simulink model "afe_abc_inv_psm_2mods"  (R2025b)
settings: Solver=ode1be  StartTime=0.0  StopTime=simlength  FixedStep=tc  MaxStep=tc
values from neighbouring files (symbols this model uses):
  n1 = 35    [voltage_islandmode_spectrum_analysis.m]    (also in voltage_spectrum_analysis.m)
undefined symbols (not defined in the file or in its folder): Adrso, afe_pwm_phase_shift_mod1, afe_pwm_phase_shift_mod2, Amplitude_U, Amplitude_V, Amplitude_W, Aresd, Bresd, Cresd, Crso, CTRPIFF_CLIP_RELEASE, dead_time_AFE, dead_time_INV, deepNEGeta, deepNEGxi, deepPOSxi, emf_fb_p, emf_fb_p_ccaller_1, emf_fb_p_ccaller_2, emf_p, emf_p_ccaller_1, emf_p_ccaller_2, end_time_LVRT, fPWM_AFE, fPWM_INV, g0_161Hz, g0_500Hz, g1_161Hz, g1_500Hz, i_grid_neg_eta_lim, i_grid_neg_eta_red_lim, i_grid_neg_xi_lim, i_grid_neg_xi_red_lim, i_grid_pos_eta_lim, i_grid_pos_eta_red_lim, ibez, id_lim, ieta_neg_ref_lim, ieta_pos_ref_lim, Igrid_phase_normalization_factor, inv_pwm_phase_shift_mod1, iq_lim, ixi_pos_ref_lim, k_frt_ref, kg, ki_afe, ki_i, ki_rc_neg_grid, ki_rc_pos_grid, ki_vs, ki_w, kp_afe, kp_i, kp_rc_neg_grid, kp_rc_pos_grid, kp_vs, kp_w, kw, l1, l2 ... (+55)
libraries: fl_lib x215, nesl_utility x107, simulink x22, cstblocks x18, threephase_inductor_lib x4, single_phase_transformer_lib x3, flexshaft_lib x1, psm x1
(part 7 of 17)

== system afe_abc_inv_psm_2mods/afe_abc_inv_psm_mod2/afe/sv_pwm/modulator1 ==
  u : Inport
  v : Inport  Port=2
  w : Inport  Port=3
  phase : Inport  Port=4
  Bus Creator : BusCreator  Inputs=3
  PWM generator : Subsystem  mask{f=fPWM_AFE, m_up=0.98, m_low=0.02, dead_time=dead_time_AFE, pos_cmd_gate=15, neg_cmd_gate=-10, polarity=1, tc=tc}
      mask prompts: f "Frequency (Hz)"; m_up "Max Input Modulation Value"; m_low "Min Input Modulation Value"; dead_time "Dead Time (s)"; pos_cmd_gate "Positive Gate Voltage (V)"; neg_cmd_gate "Negative Gate Voltage (V)"; polarity "Polarity (pu)"; tc "Sampling time"
  gate_cmds : Outport
  tag scope: TRGO_afe_module_2=global
  wires:
  PWM generator/2(gate_cmds) -> gate_cmds/1
  phase/1 -> PWM generator/2(phase)
  w/1 -> Bus Creator/3
  v/1 -> Bus Creator/2
  u/1 -> Bus Creator/1
  PWM generator/1(trgo) -> [TRGO_afe_module_2]
  Bus Creator/1 -> PWM generator/3(m_uvw())
  [time_afe_module_2] -> PWM generator/1(time_source)

== system afe_abc_inv_psm_2mods/afe_abc_inv_psm_mod2/inverter/inverter/sv_pwm ==
  duties_uvw : Inport
  Bus Selector2 : BusSelector  OutputSignals=du(k),dv(k),dw(k)
  Constant1 : Constant  Value=inv_pwm_phase_shift_mod1
  modulator1 : Subsystem
  td2tc_1 : TransferFcn  Denominator=[tc 1]
  td2tc_2 : TransferFcn  Denominator=[tc 1]
  td2tc_3 : TransferFcn  Denominator=[tc 1]
  gate_cmds : Outport
  wires:
  td2tc_2/1 -> modulator1/2(v)  "dv(t)"
  td2tc_3/1 -> modulator1/3(w)  "dw(t)"
  td2tc_1/1 -> modulator1/1(u)  "du(t)"
  duties_uvw/1 -> Bus Selector2/1
  Bus Selector2/3 -> td2tc_3/1  "<dw(k)>"
  Bus Selector2/2 -> td2tc_2/1  "<dv(k)>"
  Bus Selector2/1 -> td2tc_1/1  "<du(k)>"
  Constant1/1 -> modulator1/4(phase)
  modulator1/1(gate_cmds) -> gate_cmds/1

== system afe_abc_inv_psm_2mods/afe_abc_inv_psm_mod2/inverter/inverter/switch_1 ==
  Diode : fl_lib/Electrical/Electrical Elements/Diode  Vf=Vgamma V  Ron=Ron Ohm  Goff=1e-8 1/Ohm  i_specify=off  i_priority=None  i=0 A  i_nominal_specify=off  i_nominal_value=1  i_nominal_unit=A  v_specify=off  v_priority=None  v=0 V  v_nominal_specify=off  v_nominal_value=1  v_nominal_unit=V
  Switch : fl_lib/Electrical/Electrical Elements/Switch  R_closed=Ron Ohm  G_open=1e-8 1/Ohm  Threshold=7.5  i_specify=off  i_priority=None  i=0 A  i_nominal_specify=off  i_nominal_value=1  i_nominal_unit=A  v_specify=off  v_priority=None  v=0 V  v_nominal_specify=off  v_nominal_value=1  v_nominal_unit=V
  snubber : fl_lib/Electrical/Electrical Elements/Capacitor  c=Csnubber F  r=Rsnubber Ohm  g=0 1/Ohm  i_specify=off  i_priority=None  i=0 A  i_nominal_specify=off  i_nominal_value=1  i_nominal_unit=A  v_specify=off  v_priority=None  v=0 V  v_nominal_specify=off  v_nominal_value=1  v_nominal_unit=V  vc_specify=off  vc_priority=High  vc=0 V  vc_nominal_specify=off  vc_nominal_value=1  vc_nominal_unit=V
  G : PMIOPort  Side=Left
  C : PMIOPort  Port=2  Side=Left
  E : PMIOPort  Port=3  Side=Right
  connections:
  Diode/LConn1 -- snubber/RConn1 -- E/RConn1 -- Switch/LConn1
  Switch/RConn1 -- G/RConn1
  Diode/RConn1 -- snubber/LConn1 -- C/RConn1 -- Switch/RConn2

== system afe_abc_inv_psm_2mods/afe_abc_inv_psm_mod2/inverter/inverter/switch_2 ==
  Diode : fl_lib/Electrical/Electrical Elements/Diode  Vf=Vgamma V  Ron=Ron Ohm  Goff=1e-8 1/Ohm  i_specify=off  i_priority=None  i=0 A  i_nominal_specify=off  i_nominal_value=1  i_nominal_unit=A  v_specify=off  v_priority=None  v=0 V  v_nominal_specify=off  v_nominal_value=1  v_nominal_unit=V
  Switch : fl_lib/Electrical/Electrical Elements/Switch  R_closed=Ron Ohm  G_open=1e-8 1/Ohm  Threshold=7.5  i_specify=off  i_priority=None  i=0 A  i_nominal_specify=off  i_nominal_value=1  i_nominal_unit=A  v_specify=off  v_priority=None  v=0 V  v_nominal_specify=off  v_nominal_value=1  v_nominal_unit=V
  snubber : fl_lib/Electrical/Electrical Elements/Capacitor  c=Csnubber F  r=Rsnubber Ohm  g=0 1/Ohm  i_specify=off  i_priority=None  i=0 A  i_nominal_specify=off  i_nominal_value=1  i_nominal_unit=A  v_specify=off  v_priority=None  v=0 V  v_nominal_specify=off  v_nominal_value=1  v_nominal_unit=V  vc_specify=off  vc_priority=High  vc=0 V  vc_nominal_specify=off  vc_nominal_value=1  vc_nominal_unit=V
  G : PMIOPort  Side=Left
  C : PMIOPort  Port=2  Side=Left
  E : PMIOPort  Port=3  Side=Right
  connections:
  Switch/RConn2 -- C/RConn1 -- Diode/RConn1 -- snubber/LConn1
  Switch/RConn1 -- G/RConn1
  Diode/LConn1 -- Switch/LConn1 -- E/RConn1 -- snubber/RConn1

== system afe_abc_inv_psm_2mods/afe_abc_inv_psm_mod2/inverter/inverter/switch_3 ==
  Diode : fl_lib/Electrical/Electrical Elements/Diode  Vf=Vgamma V  Ron=Ron Ohm  Goff=1e-8 1/Ohm  i_specify=off  i_priority=None  i=0 A  i_nominal_specify=off  i_nominal_value=1  i_nominal_unit=A  v_specify=off  v_priority=None  v=0 V  v_nominal_specify=off  v_nominal_value=1  v_nominal_unit=V
  Switch : fl_lib/Electrical/Electrical Elements/Switch  R_closed=Ron Ohm  G_open=1e-8 1/Ohm  Threshold=7.5  i_specify=off  i_priority=None  i=0 A  i_nominal_specify=off  i_nominal_value=1  i_nominal_unit=A  v_specify=off  v_priority=None  v=0 V  v_nominal_specify=off  v_nominal_value=1  v_nominal_unit=V
  snubber : fl_lib/Electrical/Electrical Elements/Capacitor  c=Csnubber F  r=Rsnubber Ohm  g=0 1/Ohm  i_specify=off  i_priority=None  i=0 A  i_nominal_specify=off  i_nominal_value=1  i_nominal_unit=A  v_specify=off  v_priority=None  v=0 V  v_nominal_specify=off  v_nominal_value=1  v_nominal_unit=V  vc_specify=off  vc_priority=High  vc=0 V  vc_nominal_specify=off  vc_nominal_value=1  vc_nominal_unit=V
  G : PMIOPort  Side=Left
  C : PMIOPort  Port=2  Side=Left
  E : PMIOPort  Port=3  Side=Right
  connections:
  snubber/RConn1 -- E/RConn1 -- Switch/LConn1 -- Diode/LConn1
  Switch/RConn1 -- G/RConn1
  snubber/LConn1 -- Diode/RConn1 -- C/RConn1 -- Switch/RConn2

== system afe_abc_inv_psm_2mods/afe_abc_inv_psm_mod2/inverter/inverter/switch_4 ==
  Diode : fl_lib/Electrical/Electrical Elements/Diode  Vf=Vgamma V  Ron=Ron Ohm  Goff=1e-8 1/Ohm  i_specify=off  i_priority=None  i=0 A  i_nominal_specify=off  i_nominal_value=1  i_nominal_unit=A  v_specify=off  v_priority=None  v=0 V  v_nominal_specify=off  v_nominal_value=1  v_nominal_unit=V
  Switch : fl_lib/Electrical/Electrical Elements/Switch  R_closed=Ron Ohm  G_open=1e-8 1/Ohm  Threshold=7.5  i_specify=off  i_priority=None  i=0 A  i_nominal_specify=off  i_nominal_value=1  i_nominal_unit=A  v_specify=off  v_priority=None  v=0 V  v_nominal_specify=off  v_nominal_value=1  v_nominal_unit=V
  snubber : fl_lib/Electrical/Electrical Elements/Capacitor  c=Csnubber F  r=Rsnubber Ohm  g=0 1/Ohm  i_specify=off  i_priority=None  i=0 A  i_nominal_specify=off  i_nominal_value=1  i_nominal_unit=A  v_specify=off  v_priority=None  v=0 V  v_nominal_specify=off  v_nominal_value=1  v_nominal_unit=V  vc_specify=off  vc_priority=High  vc=0 V  vc_nominal_specify=off  vc_nominal_value=1  vc_nominal_unit=V
  G : PMIOPort  Side=Left
  C : PMIOPort  Port=2  Side=Left
  E : PMIOPort  Port=3  Side=Right
  connections:
  Switch/RConn2 -- C/RConn1 -- Diode/RConn1 -- snubber/LConn1
  Switch/RConn1 -- G/RConn1
  Diode/LConn1 -- Switch/LConn1 -- E/RConn1 -- snubber/RConn1

== system afe_abc_inv_psm_2mods/afe_abc_inv_psm_mod2/inverter/inverter/switch_5 ==
  Diode : fl_lib/Electrical/Electrical Elements/Diode  Vf=Vgamma V  Ron=Ron Ohm  Goff=1e-8 1/Ohm  i_specify=off  i_priority=None  i=0 A  i_nominal_specify=off  i_nominal_value=1  i_nominal_unit=A  v_specify=off  v_priority=None  v=0 V  v_nominal_specify=off  v_nominal_value=1  v_nominal_unit=V
  Switch : fl_lib/Electrical/Electrical Elements/Switch  R_closed=Ron Ohm  G_open=1e-8 1/Ohm  Threshold=7.5  i_specify=off  i_priority=None  i=0 A  i_nominal_specify=off  i_nominal_value=1  i_nominal_unit=A  v_specify=off  v_priority=None  v=0 V  v_nominal_specify=off  v_nominal_value=1  v_nominal_unit=V
  snubber : fl_lib/Electrical/Electrical Elements/Capacitor  c=Csnubber F  r=Rsnubber Ohm  g=0 1/Ohm  i_specify=off  i_priority=None  i=0 A  i_nominal_specify=off  i_nominal_value=1  i_nominal_unit=A  v_specify=off  v_priority=None  v=0 V  v_nominal_specify=off  v_nominal_value=1  v_nominal_unit=V  vc_specify=off  vc_priority=High  vc=0 V  vc_nominal_specify=off  vc_nominal_value=1  vc_nominal_unit=V
  G : PMIOPort  Side=Left
  C : PMIOPort  Port=2  Side=Left
  E : PMIOPort  Port=3  Side=Right
  connections:
  snubber/RConn1 -- E/RConn1 -- Switch/LConn1 -- Diode/LConn1
  Switch/RConn1 -- G/RConn1
  snubber/LConn1 -- Diode/RConn1 -- C/RConn1 -- Switch/RConn2

== system afe_abc_inv_psm_2mods/afe_abc_inv_psm_mod2/inverter/inverter/switch_6 ==
  Diode : fl_lib/Electrical/Electrical Elements/Diode  Vf=Vgamma V  Ron=Ron Ohm  Goff=1e-8 1/Ohm  i_specify=off  i_priority=None  i=0 A  i_nominal_specify=off  i_nominal_value=1  i_nominal_unit=A  v_specify=off  v_priority=None  v=0 V  v_nominal_specify=off  v_nominal_value=1  v_nominal_unit=V
  Switch : fl_lib/Electrical/Electrical Elements/Switch  R_closed=Ron Ohm  G_open=1e-8 1/Ohm  Threshold=7.5  i_specify=off  i_priority=None  i=0 A  i_nominal_specify=off  i_nominal_value=1  i_nominal_unit=A  v_specify=off  v_priority=None  v=0 V  v_nominal_specify=off  v_nominal_value=1  v_nominal_unit=V
  snubber : fl_lib/Electrical/Electrical Elements/Capacitor  c=Csnubber F  r=Rsnubber Ohm  g=0 1/Ohm  i_specify=off  i_priority=None  i=0 A  i_nominal_specify=off  i_nominal_value=1  i_nominal_unit=A  v_specify=off  v_priority=None  v=0 V  v_nominal_specify=off  v_nominal_value=1  v_nominal_unit=V  vc_specify=off  vc_priority=High  vc=0 V  vc_nominal_specify=off  vc_nominal_value=1  vc_nominal_unit=V
  G : PMIOPort  Side=Left
  C : PMIOPort  Port=2  Side=Left
  E : PMIOPort  Port=3  Side=Right
  connections:
  Switch/RConn2 -- C/RConn1 -- Diode/RConn1 -- snubber/LConn1
  Switch/RConn1 -- G/RConn1
  Diode/LConn1 -- Switch/LConn1 -- E/RConn1 -- snubber/RConn1

== system afe_abc_inv_psm_2mods/grid/grid_emulator/grid_emulator/phase_gen ==
  Constant4 : Constant  Value=omega_grid_emulator_nom
  Integrator : Integrator
  To Workspace7 : ToWorkspace  VariableName=gamma_grid_emulator_sim  SampleTime=ts_afe
      settings: MaxDataPoints=Ns_afe
  bounder1 : MATLAB Function  TreatAsAtomicUnit=on  SystemSampleTime=ts_afe
  grid_emu_phase : Outport  VectorParamsAs1DForOutWhenUnconnected=off
  tag scope: gamma_grid_emulator=global
  wires:
  bounder1/1(y) -> [gamma_grid_emulator], To Workspace7/1, grid_emu_phase/1  "grid_emu_phase"
  Constant4/1 -> Integrator/1
  Integrator/1 -> bounder1/1(u)

== system afe_abc_inv_psm_2mods/grid/grid_emulator/grid_emulator/voltage_reference ==
  grid_emu_phase : Inport
  Vxi_p : Inport  Port=2
  Vxi_n : Inport  Port=3
  Veta_n : Inport  Port=4
  Constant2 : Constant  Value=0
  Sum1 : Sum  Inputs=|++
  Sum4 : Sum  Inputs=|++
  Variant Source : VariantSource  VariantControls={enable_frt_2 == 1, enable_frt_1 == 1}
  Variant Source1 : VariantSource  VariantControls={enable_frt_2 == 1, enable_frt_1 == 1}
  Variant Source2 : VariantSource  VariantControls={enable_frt_2 == 1, enable_frt_1 == 1}
  alphabeta2abc : MATLAB Function  TreatAsAtomicUnit=on  SystemSampleTime=ts_afe
  voltage_dource_with_frt : Subsystem
  xieta2alphabeta_neg : MATLAB Function  TreatAsAtomicUnit=on  SystemSampleTime=ts_afe
  xieta2alphabeta_pos : MATLAB Function  TreatAsAtomicUnit=on  SystemSampleTime=ts_afe
  V1_ref : Outport  VectorParamsAs1DForOutWhenUnconnected=off
  V2_ref : Outport  Port=2  VectorParamsAs1DForOutWhenUnconnected=off
  V3_ref : Outport  Port=3  VectorParamsAs1DForOutWhenUnconnected=off
  wires:
  xieta2alphabeta_pos/1(alpha) -> Sum1/1
  Sum1/1 -> alphabeta2abc/1(alpha)
  xieta2alphabeta_pos/2(beta) -> Sum4/1
  Sum4/1 -> alphabeta2abc/2(beta)
  xieta2alphabeta_neg/1(alpha) -> Sum1/2
  xieta2alphabeta_neg/2(beta) -> Sum4/2
  grid_emu_phase/1 -> voltage_dource_with_frt/1(gamma), xieta2alphabeta_neg/3(gamma), xieta2alphabeta_pos/3(gamma)
  Vxi_p/1 -> xieta2alphabeta_pos/1(xi)
  Constant2/1 -> xieta2alphabeta_pos/2(eta)
  Vxi_n/1 -> xieta2alphabeta_neg/1(xi)
  Veta_n/1 -> xieta2alphabeta_neg/2(eta)
  Variant Source/1 -> V1_ref/1
  alphabeta2abc/1(a) -> [V1_ref_xieta]
  alphabeta2abc/2(b) -> [V2_ref_xieta]
  alphabeta2abc/3(c) -> [V3_ref_xieta]
  voltage_dource_with_frt/3(vn_eta) -> [V3_ref_abc]
  voltage_dource_with_frt/2(vn_xi) -> [V2_ref_abc]
  voltage_dource_with_frt/1(vp_xi) -> [V1_ref_abc]
  [V1_ref_xieta] -> Variant Source/1
  [V1_ref_abc] -> Variant Source/2
  Variant Source1/1 -> V2_ref/1
  [V2_ref_xieta] -> Variant Source1/1
  [V2_ref_abc] -> Variant Source1/2
  Variant Source2/1 -> V3_ref/1
  [V3_ref_abc] -> Variant Source2/2
  [V3_ref_xieta] -> Variant Source2/1

== system afe_abc_inv_psm_2mods/grid/grid_emulator/grid_emulator/voltage_source ==
  Add10 : Sum  Inputs=+-+
  Add11 : Sum  Inputs=+-+
  Add12 : Sum  Inputs=+-+
  Constant : Constant  Value=vp_xi_pu
  Constant1 : Constant  Value=vn_xi_pu
  Constant2 : Constant  Value=vn_eta_pu
  Gain1 : Gain  Gain=V_phase_normalization_factor
  Gain2 : Gain  Gain=ugrid_factor
  Gain3 : Gain  Gain=ugrid_factor
  Gain4 : Gain  Gain=ugrid_factor
  Gain7 : Gain  Gain=V_phase_normalization_factor
  Gain8 : Gain  Gain=V_phase_normalization_factor
  LTI System1 : cstblocks/LTI System  sys=LVRT_flt_ss_c  IC=[0]  PadeOrder=0
  LTI System2 : cstblocks/LTI System  sys=LVRT_flt_ss_c  IC=[0]  PadeOrder=0
  LTI System3 : cstblocks/LTI System  sys=LVRT_flt_ss_c  IC=[]  PadeOrder=0
  LTI System4 : cstblocks/LTI System  sys=LVRT_flt_ss_c  IC=[]  PadeOrder=0
  LTI System5 : cstblocks/LTI System  sys=LVRT_flt_ss_c  IC=[]  PadeOrder=0
  LTI System6 : cstblocks/LTI System  sys=LVRT_flt_ss_c  IC=[0]  PadeOrder=0
  Rate Limiter{1..9} (9 alike) : RateLimiter  RisingSlewLimit=Vemu_ref_norm/t_ramp  FallingSlewLimit=-Vemu_ref_norm/t_ramp  SampleTimeMode=inherited
  Step10 : Step  Time=end_time_LVRT  After=vp_xi_pu*deepPOSxi  SampleTime=0
  Step11 : Step  Time=0  After=vn_eta_pu  SampleTime=0
  Step12 : Step  Time=start_time_LVRT  After=deepNEGeta  SampleTime=0
  Step13 : Step  Time=end_time_LVRT  After=deepNEGeta  SampleTime=0
  Step5 : Step  Time=0  After=vn_xi_pu  SampleTime=0
  Step6 : Step  Time=start_time_LVRT  After=deepNEGxi  SampleTime=0
  Step7 : Step  Time=end_time_LVRT  After=deepNEGxi  SampleTime=0
  Step8 : Step  Time=0  After=vp_xi_pu  SampleTime=0
  Step9 : Step  Time=start_time_LVRT  After=vp_xi_pu*deepPOSxi  SampleTime=0
  vp_xi : Outport  VectorParamsAs1DForOutWhenUnconnected=off
  vn_xi : Outport  Port=2  VectorParamsAs1DForOutWhenUnconnected=off
  vn_eta : Outport  Port=3  VectorParamsAs1DForOutWhenUnconnected=off
  wires:
  LTI System3/1 -> Gain7/1
  LTI System4/1 -> Gain8/1
  Gain7/1 -> Gain2/1
  Gain8/1 -> Gain3/1
  Gain1/1 -> Gain4/1
  LTI System5/1 -> Gain1/1
  Gain2/1 -> vp_xi/1
  Gain3/1 -> vn_xi/1
  Gain4/1 -> vn_eta/1
  LTI System6/1 -> LTI System5/1
  LTI System1/1 -> LTI System4/1
  LTI System2/1 -> LTI System3/1
  Rate Limiter2/1 -> Add11/3
  Add12/1 -> LTI System6/1
  Step7/1 -> Rate Limiter6/1
  Step6/1 -> Rate Limiter5/1
  Rate Limiter5/1 -> Add10/2
  Step5/1 -> Rate Limiter4/1
  Add11/1 -> LTI System2/1
  Rate Limiter7/1 -> Add12/1
  Step8/1 -> Rate Limiter3/1
  Step12/1 -> Rate Limiter8/1
  Step11/1 -> Rate Limiter7/1
  Rate Limiter1/1 -> Add11/2
  Step9/1 -> Rate Limiter1/1
  Rate Limiter3/1 -> Add11/1
  Rate Limiter8/1 -> Add12/2
  Rate Limiter9/1 -> Add12/3
  Rate Limiter4/1 -> Add10/1
  Rate Limiter6/1 -> Add10/3
  Step10/1 -> Rate Limiter2/1
  Add10/1 -> LTI System1/1
  Step13/1 -> Rate Limiter9/1

== system afe_abc_inv_psm_2mods/afe_abc_inv_psm_mod1/AFE_control/afe_control/FRT-VDE4110/FRT-Detection ==
  red_dyn_enabled : Inport
  Abs : Abs  SaturateOnIntegerOverflow=off
  Abs1 : Abs  SaturateOnIntegerOverflow=off
  LVRT_detector : MATLAB Function  TreatAsAtomicUnit=on
  Step1 : Step  Time=0.025  Before=1  After=0
  Step3 : Step  Time=settle_time
  dvxi_n/dt : Subsystem
  dvxi_p/dt : Subsystem
  frt_detection_inputs : Scope  NumInputPorts=6
      settings: ActiveDisplayYMinimum=-0.12991  ActiveDisplayYMaximum=1.13961  DataLoggingVariableName=ScopeData2
  frt_exceeded : Outport
  frt_state : Outport  Port=2
  red_dyn_active : Outport  Port=3
  frt_active : Outport  Port=4
  pwr_lim_enable : Outport  Port=5
  wires:
  [v_grid_neg_xi_avg_mod1] -> LVRT_detector/2(vxi_n), frt_detection_inputs/2, dvxi_n/dt/1(x)  "v_grid_neg_xi_avg"
  [v_grid_pos_xi_avg_mod1] -> LVRT_detector/1(vxi_p), frt_detection_inputs/1, dvxi_p/dt/1(x)  "v_grid_pos_xi_avg"
  [v_grid_neg_eta_avg_mod1] -> LVRT_detector/3(veta_n), frt_detection_inputs/3  "v_grid_neg_eta_avg"
  Step3/1 -> frt_detection_inputs/6, LVRT_detector/6(enable)  "enable"
  dvxi_p/dt/1(xdot_hat) -> Abs/1
  LVRT_detector/1(pwr_lim_enable) -> pwr_lim_enable/1  "pwr_lim_enable"
  dvxi_n/dt/1(xdot_hat) -> Abs1/1
  Step1/1 -> LVRT_detector/8(reset)
  red_dyn_enabled/1 -> LVRT_detector/7(red_dyn_enabled)
  LVRT_detector/2(frt_exceeded) -> frt_exceeded/1  "lvrt_exceeded"
  LVRT_detector/5(red_dyn_active) -> red_dyn_active/1
  LVRT_detector/4(frt_state) -> frt_state/1
  LVRT_detector/3(frt_active) -> frt_active/1
  Abs/1 -> frt_detection_inputs/4, LVRT_detector/4(vxi_p_dot)  "vxi_pos_dot"
  Abs1/1 -> frt_detection_inputs/5, LVRT_detector/5(vxi_n_dot)  "vxi_neg_dot"

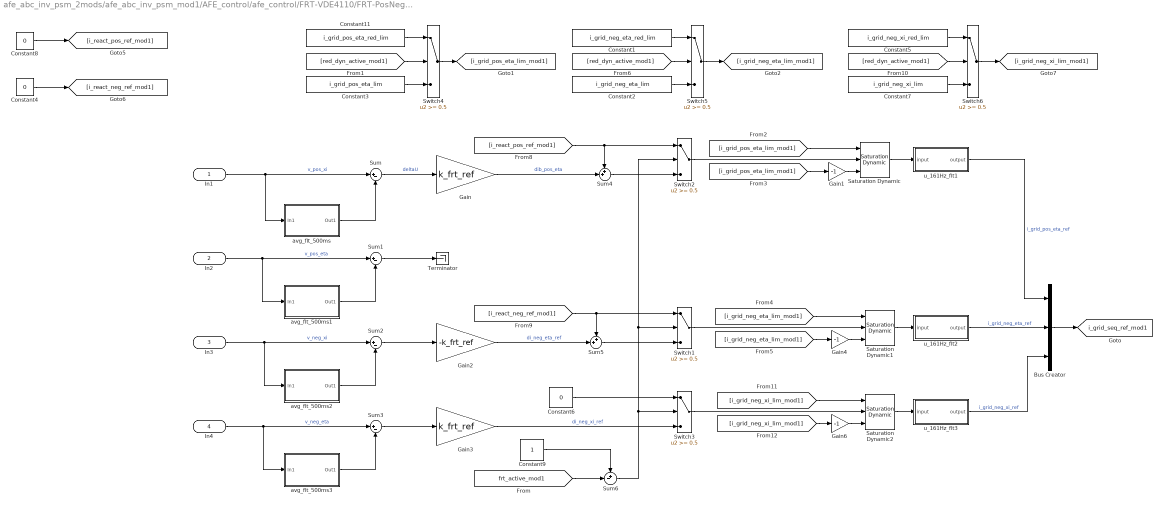
== system afe_abc_inv_psm_2mods/afe_abc_inv_psm_mod1/AFE_control/afe_control/FRT-VDE4110/FRT-PosNegReactiveCurrentReferences ==
  In1 : Inport
  In2 : Inport  Port=2
  In3 : Inport  Port=3
  In4 : Inport  Port=4
  Bus Creator : BusCreator  Inputs=3
  Constant1 : Constant  Value=i_grid_neg_eta_red_lim
  Constant11 : Constant  Value=i_grid_pos_eta_red_lim
  Constant2 : Constant  Value=i_grid_neg_eta_lim
  Constant3 : Constant  Value=i_grid_pos_eta_lim
  Constant4 : Constant  Value=0
  Constant5 : Constant  Value=i_grid_neg_xi_red_lim
  Constant6 : Constant  Value=0
  Constant7 : Constant  Value=i_grid_neg_xi_lim
  Constant8 : Constant  Value=0
  Constant9 : Constant
  Gain : Gain  Gain=k_frt_ref
  Gain1 : Gain  Gain=-1
  Gain2 : Gain  Gain=-k_frt_ref
  Gain3 : Gain  Gain=k_frt_ref
  Gain4 : Gain  Gain=-1
  Gain6 : Gain  Gain=-1
  Saturation Dynamic : simulink/Discontinuities/Saturation Dynamic  OutMin=[]  OutMax=[]  OutDataTypeStr=Inherit: Same as second input  OutDataType=fixdt(1, 16)  OutScaling=2^-10  DoSatur=off
  Saturation Dynamic1 : simulink/Discontinuities/Saturation Dynamic  OutMin=[]  OutMax=[]  OutDataTypeStr=Inherit: Same as second input  OutDataType=fixdt(1, 16)  OutScaling=2^-10  DoSatur=off
  Saturation Dynamic2 : simulink/Discontinuities/Saturation Dynamic  OutMin=[]  OutMax=[]  OutDataTypeStr=Inherit: Same as second input  OutDataType=fixdt(1, 16)  OutScaling=2^-10  DoSatur=off
  Sum{,1..3} (4 alike) : Sum  Inputs=|+-
  Sum4 : Sum  Inputs=++|
  Sum5 : Sum  Inputs=++|
  Sum6 : Sum  Inputs=+-|
  Switch{1..6} (6 alike) : Switch  Threshold=0.5  SaturateOnIntegerOverflow=off  InputSameDT=off
  Terminator : Terminator
  avg_flt_500ms : Subsystem
  avg_flt_500ms1 : Subsystem
  avg_flt_500ms2 : Subsystem
  avg_flt_500ms3 : Subsystem
  u_161Hz_flt1 : Subsystem
  u_161Hz_flt2 : Subsystem
  u_161Hz_flt3 : Subsystem
  tag scope: i_grid_seq_ref_mod1=global
  wires:
  In1/1 -> avg_flt_500ms/1(In1), Sum/1  "v_pos_xi"
  avg_flt_500ms/1(Out1) -> Sum/2
  Sum/1 -> Gain/1  "deltaU"
  Sum1/1 -> Terminator/1
  avg_flt_500ms1/1(Out1) -> Sum1/2
  In2/1 -> avg_flt_500ms1/1(In1), Sum1/1  "v_pos_eta"
  avg_flt_500ms3/1(Out1) -> Sum3/2
  Sum2/1 -> Gain2/1
  In3/1 -> avg_flt_500ms2/1(In1), Sum2/1  "v_neg_xi"
  avg_flt_500ms2/1(Out1) -> Sum2/2
  In4/1 -> avg_flt_500ms3/1(In1), Sum3/1  "v_neg_eta"
  Bus Creator/1 -> [i_grid_seq_ref_mod1]
  Gain/1 -> Sum4/2  "dib_pos_eta"
  [i_react_pos_ref_mod1] -> Switch2/1, Sum4/1
  Sum4/1 -> Switch2/3
  Switch2/1 -> Saturation Dynamic/2
  Saturation Dynamic/1 -> u_161Hz_flt1/1(input)
  Constant6/1 -> Switch3/1
  Gain3/1 -> Switch3/3  "di_neg_xi_ref"
  Sum6/1 -> Switch1/2, Switch2/2, Switch3/2
  Sum3/1 -> Gain3/1
  Gain2/1 -> Sum5/2  "di_neg_eta_ref"
  Sum5/1 -> Switch1/3
  [i_react_neg_ref_mod1] -> Switch1/1, Sum5/1
  Switch4/1 -> [i_grid_pos_eta_lim_mod1]
  [red_dyn_active_mod1] -> Switch4/2
  Constant3/1 -> Switch4/3
  Constant11/1 -> Switch4/1
  [i_grid_pos_eta_lim_mod1] -> Saturation Dynamic/1
  [i_grid_pos_eta_lim_mod1] -> Gain1/1
  Gain1/1 -> Saturation Dynamic/3
  Saturation Dynamic2/1 -> u_161Hz_flt3/1(input)
  Switch3/1 -> Saturation Dynamic2/2
  [i_grid_neg_xi_lim_mod1] -> Saturation Dynamic2/1
  [i_grid_neg_xi_lim_mod1] -> Gain6/1
  Gain4/1 -> Saturation Dynamic1/3
  [i_grid_neg_eta_lim_mod1] -> Gain4/1
  [i_grid_neg_eta_lim_mod1] -> Saturation Dynamic1/1
  Switch1/1 -> Saturation Dynamic1/2
  Saturation Dynamic1/1 -> u_161Hz_flt2/1(input)
  [red_dyn_active_mod1] -> Switch5/2
  Constant2/1 -> Switch5/3
  Constant1/1 -> Switch5/1
  Switch5/1 -> [i_grid_neg_eta_lim_mod1]
  Constant4/1 -> [i_react_neg_ref_mod1]
  Constant8/1 -> [i_react_pos_ref_mod1]
  Constant7/1 -> Switch6/3
  Switch6/1 -> [i_grid_neg_xi_lim_mod1]
  Constant5/1 -> Switch6/1
  [red_dyn_active_mod1] -> Switch6/2
  Gain6/1 -> Saturation Dynamic2/3
  u_161Hz_flt2/1(output) -> Bus Creator/2  "i_grid_neg_eta_ref"
  u_161Hz_flt3/1(output) -> Bus Creator/3  "i_grid_neg_xi_ref"
  u_161Hz_flt1/1(output) -> Bus Creator/1  "i_grid_pos_eta_ref"
  [frt_active_mod1] -> Sum6/2
  Constant9/1 -> Sum6/1

== system afe_abc_inv_psm_2mods/afe_abc_inv_psm_mod1/AFE_control/afe_control/current_ctrl/Inner Loop Current Control ==
  In1 : Inport
  is_abc : Inport  Port=2
  -1<x<1 : Saturate  UpperLimit=1  LowerLimit=-1
  Add : Sum
  Bus Creator1 : BusCreator  Inputs=2
  "Current-Control, Phase a" : Subsystem
  "Current-Control, Phase b" : Subsystem
  "Current-Control, Phase c" : Subsystem
  Demux1 : Demux  Outputs=3
  MATLAB Function : MATLAB Function  TreatAsAtomicUnit=on
  Mux : Mux  Inputs=3
  Selector : Selector  InputPortWidth=3  IndexOptions=Index vector (dialog)  Indices=[1]  OutputSizes=1
  Selector1 : Selector  InputPortWidth=3  IndexOptions=Index vector (dialog)  Indices=[1]  OutputSizes=1
  Selector2 : Selector  InputPortWidth=3  IndexOptions=Index vector (dialog)  Indices=[2]  OutputSizes=1
  Selector3 : Selector  InputPortWidth=3  IndexOptions=Index vector (dialog)  Indices=[2]  OutputSizes=1
  Selector4 : Selector  InputPortWidth=3  IndexOptions=Index vector (dialog)  Indices=[3]  OutputSizes=1
  Selector5 : Selector  InputPortWidth=3  IndexOptions=Index vector (dialog)  Indices=[3]  OutputSizes=1
  To Workspace1 : ToWorkspace  VariableName=isa_ref_sim_mod1  SampleTime=-1
      settings: MaxDataPoints=Ns_afe
  To Workspace2 : ToWorkspace  VariableName=isa_sim_mod1  SampleTime=-1
      settings: MaxDataPoints=Ns_afe
  To Workspace3 : ToWorkspace  VariableName=isb_ref_sim_mod1  SampleTime=-1
      settings: MaxDataPoints=Ns_afe
  To Workspace4 : ToWorkspace  VariableName=isb_sim_mod1  SampleTime=-1
      settings: MaxDataPoints=Ns_afe
  To Workspace5 : ToWorkspace  VariableName=isc_ref_sim_mod1  SampleTime=-1
      settings: MaxDataPoints=Ns_afe
  To Workspace6 : ToWorkspace  VariableName=isc_sim_mod1  SampleTime=-1
      settings: MaxDataPoints=Ns_afe
  Unit Delay1 : UnitDelay  SampleTime=-1  HasFrameUpgradeWarning=on
  Unit Delay2 : UnitDelay  SampleTime=-1  HasFrameUpgradeWarning=on
  Unit Delay3 : UnitDelay  SampleTime=-1  HasFrameUpgradeWarning=on
  afe_ictrl_out/afe_ictrl_ff : Scope  NumInputPorts=2
      settings: ActiveDisplayYMinimum=-1.2844276731305864  ActiveDisplayYMaximum=1.2966894715372321  DataLoggingVariableName=ScopeData4
  isa_ref/isa : Scope  NumInputPorts=2
      settings: ActiveDisplayYMinimum=-1.06078125  ActiveDisplayYMaximum=1.00328125
  isb_ref/isb : Scope  NumInputPorts=2
      settings: ActiveDisplayYMinimum=-1.080322265625  ActiveDisplayYMaximum=1.007080078125  DataLoggingVariableName=ScopeData2
  isc_ref/isc : Scope  NumInputPorts=2
      settings: ActiveDisplayYMinimum=-1.005859375  ActiveDisplayYMaximum=1.0791015625  DataLoggingVariableName=ScopeData3
  uab : Outport  VectorParamsAs1DForOutWhenUnconnected=off
  wires:
  In1/1 -> Selector4/1, Selector2/1, Selector/1  "id_abc_ref"
  is_abc/1 -> Selector5/1, Selector3/1, Selector1/1  "id_abc"
  Add/1 -> -1<x<1/1  "v_abc"
  Selector/1 -> isa_ref/isa/1, [isa_ref_mod1], "Current-Control, Phase a"/1(In1)  "isa_ref"
  Selector1/1 -> [isa_mod1], isa_ref/isa/2, "Current-Control, Phase a"/2(In2)  "isa"
  Selector2/1 -> [isb_ref_mod1], isb_ref/isb/1, "Current-Control, Phase b"/1(In1)  "isb_ref"
  Selector3/1 -> [isb_mod1], isb_ref/isb/2, "Current-Control, Phase b"/2(In2)  "isb"
  Selector4/1 -> isc_ref/isc/1, [isc_ref_mod1], "Current-Control, Phase c"/1(In1)  "isc_ref"
  Selector5/1 -> isc_ref/isc/2, [isc_mod1], "Current-Control, Phase c"/2(In2)  "isc"
  "Current-Control, Phase a"/1(Out1) -> Mux/1  "v_a"
  "Current-Control, Phase b"/1(Out1) -> Mux/2  "v_b"
  "Current-Control, Phase c"/1(Out1) -> Mux/3  "v_c"
  Mux/1 -> Add/1, afe_ictrl_out/afe_ictrl_ff/1  "v_abc"
  Demux1/3 -> MATLAB Function/3(c)  "v_c"
  MATLAB Function/1(alpha) -> Unit Delay2/1  "u_alpha"
  Unit Delay3/1 -> Bus Creator1/2  "ubeta_afe"
  Demux1/2 -> MATLAB Function/2(b)  "v_b"
  MATLAB Function/2(beta) -> Unit Delay3/1  "u_beta"
  Demux1/1 -> MATLAB Function/1(a)  "v_a"
  Unit Delay2/1 -> Bus Creator1/1  "ualpha_afe"
  Bus Creator1/1 -> uab/1
  -1<x<1/1 -> Demux1/1  "v_abc"
  Unit Delay1/1 -> afe_ictrl_out/afe_ictrl_ff/2  "v_grid_ff_abc_mod1"
  [v_grid_ff_abc_mod1] -> Unit Delay1/1
  [isa_ref_mod1] -> To Workspace1/1
  [isa_mod1] -> To Workspace2/1
  [isb_mod1] -> To Workspace4/1
  [isb_ref_mod1] -> To Workspace3/1
  [isc_ref_mod1] -> To Workspace5/1
  [isc_mod1] -> To Workspace6/1

== system afe_abc_inv_psm_2mods/afe_abc_inv_psm_mod1/AFE_control/afe_control/current_ctrl/current_transformation ==
  is_a_pu : Inport
  is_b_pu : Inport  Port=2
  is_c_pu : Inport  Port=3
  alphabeta2xieta : MATLAB Function  TreatAsAtomicUnit=on
  uvw2alphabeta : MATLAB Function  TreatAsAtomicUnit=on
  tag scope: id_eta_pu_mod1=global, id_xi_pu_mod1=global
  wires:
  is_c_pu/1 -> uvw2alphabeta/3(w)
  alphabeta2xieta/2(eta) -> [id_eta_pu_mod1]  "ieta_pu"
  alphabeta2xieta/1(xi) -> [id_xi_pu_mod1]  "ixi_pu"
  is_b_pu/1 -> uvw2alphabeta/2(v)
  uvw2alphabeta/2(beta) -> alphabeta2xieta/2(beta)  "ibeta_pu"
  uvw2alphabeta/1(alpha) -> alphabeta2xieta/1(alpha)  "ialpha_pu"
  [gamma_grid_pll_mod1] -> alphabeta2xieta/3(gamma)
  is_a_pu/1 -> uvw2alphabeta/1(u)

== system afe_abc_inv_psm_2mods/afe_abc_inv_psm_mod1/AFE_control/afe_control/current_ctrl/xieta2abc ==
  pos_xi : Inport
  pos_eta : Inport  Port=2
  neg_xi : Inport  Port=3
  neg_eta : Inport  Port=4
  gamma : Inport  Port=5
  MATLAB Function2 : MATLAB Function  TreatAsAtomicUnit=on
  Mux : Mux  Inputs=3
  Negative Sequence : MATLAB Function  TreatAsAtomicUnit=on
  Positive Sequence : MATLAB Function  TreatAsAtomicUnit=on
  Sum : Sum  Inputs=|++
  Sum1 : Sum  Inputs=|++
  i_abc : Outport
  wires:
  neg_eta/1 -> Negative Sequence/2(eta)
  MATLAB Function2/1(a) -> Mux/1  "i_a"
  Positive Sequence/2(beta) -> Sum1/1
  Sum/1 -> MATLAB Function2/1(alpha)
  gamma/1 -> Negative Sequence/3(gamma), Positive Sequence/3(gamma)
  MATLAB Function2/3(c) -> Mux/3  "i_c"
  Negative Sequence/1(alpha) -> Sum/2
  Positive Sequence/1(alpha) -> Sum/1
  Negative Sequence/2(beta) -> Sum1/2
  MATLAB Function2/2(b) -> Mux/2  "i_b"
  Sum1/1 -> MATLAB Function2/2(beta)
  neg_xi/1 -> Negative Sequence/1(xi)
  pos_xi/1 -> Positive Sequence/1(xi)
  pos_eta/1 -> Positive Sequence/2(eta)
  Mux/1 -> i_abc/1  "i_abc"

== system afe_abc_inv_psm_2mods/afe_abc_inv_psm_mod1/AFE_control/afe_control/grid_current_sequences_and_reactive_pwr_ctrl/current_sequence_avg ==
  i_grid_pos_xi : Inport
  i_grid_pos_eta : Inport  Port=2
  i_grid_neg_xi : Inport  Port=3
  i_grid_neg_eta : Inport  Port=4
  Variant Source{,1..3} (4 alike) : VariantSource  VariantControls={use_moving_average_from_ccaller_mod1 == 1, use_moving_average_from_ccaller_mod1 == 0}
  average_filter_ccaller : Subsystem
  average_filter_simulink : Subsystem
  i_grid_pos_xi_avg : Outport
  i_grid_pos_eta_avg : Outport  Port=2
  i_grid_neg_xi_avg : Outport  Port=3
  i_grid_neg_eta_avg : Outport  Port=4
  wires:
  i_grid_pos_xi/1 -> average_filter_simulink/1(i_grid_pos_xi), average_filter_ccaller/1(i_grid_pos_xi)
  i_grid_pos_eta/1 -> average_filter_simulink/2(i_grid_pos_eta), average_filter_ccaller/2(i_grid_pos_eta)
  i_grid_neg_xi/1 -> average_filter_simulink/3(i_grid_neg_xi), average_filter_ccaller/3(i_grid_neg_xi)
  i_grid_neg_eta/1 -> average_filter_simulink/4(i_grid_neg_eta), average_filter_ccaller/4(i_grid_neg_eta)
  Variant Source/1 -> i_grid_pos_xi_avg/1
  Variant Source3/1 -> i_grid_neg_eta_avg/1
  Variant Source2/1 -> i_grid_neg_xi_avg/1
  Variant Source1/1 -> i_grid_pos_eta_avg/1
  average_filter_ccaller/1(i_grid_pos_xi_avg) -> Variant Source/1
  average_filter_simulink/1(i_grid_pos_xi_avg) -> Variant Source/2
  average_filter_simulink/2(i_grid_pos_eta_avg) -> Variant Source1/2
  average_filter_simulink/3(i_grid_neg_xi_avg) -> Variant Source2/2
  average_filter_simulink/4(i_grid_neg_eta_avg) -> Variant Source3/2
  average_filter_ccaller/2(i_grid_pos_eta_avg) -> Variant Source1/1
  average_filter_ccaller/3(i_grid_neg_xi_avg) -> Variant Source2/1
  average_filter_ccaller/4(i_grid_neg_eta_avg) -> Variant Source3/1

== system afe_abc_inv_psm_2mods/afe_abc_inv_psm_mod1/AFE_control/afe_control/grid_current_sequences_and_reactive_pwr_ctrl/grid_current_sampling_and_alpha_beta_transformation ==
  ig_abc : Inport
  i_abc2alphabeta : MATLAB Function  TreatAsAtomicUnit=on
  i_grid_alpha : Outport
  i_grid_beta : Outport  Port=2
  wires:
  i_abc2alphabeta/2(beta) -> i_grid_beta/1  "i_grid_beta"
  i_abc2alphabeta/1(alpha) -> i_grid_alpha/1  "i_grid_alpha"
  ig_abc/1 -> i_abc2alphabeta/1(i_abc)

== system afe_abc_inv_psm_2mods/afe_abc_inv_psm_mod1/AFE_control/afe_control/grid_current_sequences_and_reactive_pwr_ctrl/i_alphabeta2xieta ==
  alpha : Inport
  beta : Inport  Port=2
  gamma : Inport  Port=3
  MATLAB Function : MATLAB Function  TreatAsAtomicUnit=on
  MATLAB Function1 : MATLAB Function  TreatAsAtomicUnit=on
  xi : Outport
  v_grid_pos_eta : Outport  Port=2
  v_grid_neg_xi : Outport  Port=3
  e : Outport  Port=4
  wires:
  alpha/1 -> MATLAB Function1/1(alpha), MATLAB Function/1(alpha)  "i_grid_alpha"
  beta/1 -> MATLAB Function1/2(beta), MATLAB Function/2(beta)  "i_grid_beta"
  gamma/1 -> MATLAB Function1/3(gamma), MATLAB Function/3(gamma)  "gamma_grid"
  MATLAB Function/2(eta) -> v_grid_pos_eta/1  "i_grid_pos_eta"
  MATLAB Function1/1(xi) -> v_grid_neg_xi/1  "i_grid_neg_xi"
  MATLAB Function1/2(eta) -> e/1  "i_grid_neg_eta"
  MATLAB Function/1(xi) -> xi/1  "i_grid_pos_xi"

== system afe_abc_inv_psm_2mods/afe_abc_inv_psm_mod1/AFE_control/afe_control/grid_current_sequences_and_reactive_pwr_ctrl/sequences_current_control ==
  i_pos_xi : Inport
  i_pos_eta : Inport  Port=2
  i_neg_xi : Inport  Port=3
  i_neg_eta : Inport  Port=4
  Bus Selector : BusSelector  OutputSignals=i_grid_pos_eta_ref,i_grid_neg_eta_ref,i_grid_neg_xi_ref
  Gain : Gain  Gain=-1
  Gain1 : Gain  Gain=-1
  Gain2 : Gain  Gain=-1
  Negative-Seq. eta-Control : Subsystem
  Negative-Seq. xi-Control : Subsystem
  Positive-Seq. eta-Control : Subsystem
  Sum : Sum  Inputs=|+-
  Sum1 : Sum  Inputs=|+-
  Sum2 : Sum  Inputs=|+-
  Terminator : Terminator
  i_neg_eta_ref/i_neg_eta : Scope  NumInputPorts=2
      settings: ActiveDisplayYMinimum=-0.0786294096145648  ActiveDisplayYMaximum=0.079467268368625582  DataLoggingVariableName=ScopeData6
  i_neg_xi_ref/i_neg_xi : Scope  NumInputPorts=2
      settings: ActiveDisplayYMinimum=-0.093272384387596066  ActiveDisplayYMaximum=0.21232485707584112  DataLoggingVariableName=ScopeData7
  i_pos_eta_ref/i_pos_eta : Scope  NumInputPorts=2
      settings: ActiveDisplayYMinimum=-0.13263870980821479  ActiveDisplayYMaximum=0.34001616382199712  DataLoggingVariableName=ScopeData5
  tag scope: i_stack_neg_eta_ref_mod1=global, i_stack_neg_xi_ref_mod1=global, i_stack_pos_eta_ref_mod1=global
  wires:
  i_pos_xi/1 -> Terminator/1
  [i_grid_seq_ref_mod1] -> Bus Selector/1
  Bus Selector/1 -> i_pos_eta_ref/i_pos_eta/1, Sum/1  "<i_grid_pos_eta_ref>"
  Bus Selector/2 -> Sum1/1, i_neg_eta_ref/i_neg_eta/1  "<i_grid_neg_eta_ref>"
  Bus Selector/3 -> i_neg_xi_ref/i_neg_xi/1, Sum2/1  "<i_grid_neg_xi_ref>"
  Sum2/1 -> Gain2/1
  Sum1/1 -> Gain1/1
  Sum/1 -> Gain/1
  i_pos_eta/1 -> i_pos_eta_ref/i_pos_eta/2, Sum/2  "i_pos_eta"
  i_neg_eta/1 -> Sum1/2, i_neg_eta_ref/i_neg_eta/2  "i_neg_eta"
  i_neg_xi/1 -> i_neg_xi_ref/i_neg_xi/2, Sum2/2  "i_neg_xi"
  Gain/1 -> Positive-Seq. eta-Control/2(e)
  Gain1/1 -> Negative-Seq. eta-Control/2(e)
  Gain2/1 -> Negative-Seq. xi-Control/2(e)
  Positive-Seq. eta-Control/1(u) -> [i_stack_pos_eta_ref_mod1]
  Negative-Seq. eta-Control/1(u) -> [i_stack_neg_eta_ref_mod1]
  Negative-Seq. xi-Control/1(u) -> [i_stack_neg_xi_ref_mod1]

== system afe_abc_inv_psm_2mods/afe_abc_inv_psm_mod1/AFE_control/afe_control/grid_voltage_phase_lock_loops/DDSRF-PLL ==
  ug_abc_pu : Inport
  pll_stageA : Subsystem
  pll_stageB : Subsystem
  gamma_grid_ddsrf_pll : Outport
  omega_grid_ddsrf_pll : Outport  Port=2
  wires:
  pll_stageB/1(gamma_grid_ddsrf_pll) -> pll_stageA/1(gamma_grid), gamma_grid_ddsrf_pll/1
  pll_stageA/2(u_grid_pos_eta) -> pll_stageB/2(u_grid_pos_eta)  "u_grid_pos_eta"
  pll_stageA/1(u_grid_pos_xi) -> pll_stageB/1(u_grid_pos_xi)  "u_grid_pos_xi"
  pll_stageB/2(omega_grid_ddsrf_pll) -> omega_grid_ddsrf_pll/1
  ug_abc_pu/1 -> pll_stageA/2(ug_abc_pu)

== system afe_abc_inv_psm_2mods/afe_abc_inv_psm_mod1/AFE_control/afe_control/grid_voltage_phase_lock_loops/dq_pll ==
  ug_abc_pu : Inport
  pll_stageA : Subsystem
  pll_stageB : Subsystem
  gamma_grid_dqpll : Outport
  omega_grid_dqpll : Outport  Port=2
  wires:
  pll_stageA/2(u_grid_pos_eta) -> pll_stageB/2(u_grid_pos_eta)  "u_grid_pos_eta"
  pll_stageB/1(gamma_grid_pll) -> gamma_grid_dqpll/1, pll_stageA/1(gamma_grid)
  pll_stageA/1(u_grid_pos_xi) -> pll_stageB/1(u_grid_pos_xi)  "u_grid_pos_xi"
  pll_stageB/2(omega_grid_pll) -> omega_grid_dqpll/1
  ug_abc_pu/1 -> pll_stageA/2(ug_abc)

== system afe_abc_inv_psm_2mods/afe_abc_inv_psm_mod1/AFE_control/afe_control/grid_voltage_phase_lock_loops/dq_pll_ccaller ==
  ug_abc_pu : Inport
  Bus Selector : BusSelector  OutputSignals=omega_pu_hat,gamma_hat,u_grid_xi,u_grid_eta,dqpll_pll_state
  C Caller : CCaller  FunctionName=dqpll_grid_process_simulink  PortSpecificationStruct="%)30     .    N H   8    (     @         %    \"     8    !     0         %  0 \"0    $    _    07)G3F%M90  4&]R=$YA;64 4V-O<&4     26YD97@     5'EP90      4VEZ90      27-';&]B86P   X    P    !@    @    $          4    (     0    ,    !         !   P!O=70 #@   #     &    \"     0         !0    @    !     P    $         $  # &]U=  .    .     8    (    !          %    \"     $    &     0         0   ...(+3319 chars)"
  Constant : Constant  Value=ts_afe
  Data Type Conversion{1..2,4..5} (4 alike) : DataTypeConversion  OutDataTypeStr=single  SaturateOnIntegerOverflow=off  RndMeth=Floor
  Data Type Conversion{6..10} (5 alike) : DataTypeConversion  OutDataTypeStr=double  SaturateOnIntegerOverflow=off  RndMeth=Floor
  Data Type Conversion3 : DataTypeConversion  OutDataTypeStr=uint8  SaturateOnIntegerOverflow=off  RndMeth=Floor
  Demux : Demux  Outputs=3
  Quantizer1 : Quantizer  QuantizationInterval=adc_quantization
  Quantizer2 : Quantizer  QuantizationInterval=adc_quantization
  Quantizer4 : Quantizer  QuantizationInterval=adc_quantization
  Step : Step  Time=0.01  Before=1  After=0
  Unit Delay1 : UnitDelay  SampleTime=-1  HasFrameUpgradeWarning=on
  Unit Delay2 : UnitDelay  SampleTime=-1  HasFrameUpgradeWarning=on
  Unit Delay3 : UnitDelay  SampleTime=-1  HasFrameUpgradeWarning=on
  first_harmonic_tracker : Scope  NumInputPorts=3
      settings: ActiveDisplayYMinimum=-1.7184470891952515  ActiveDisplayYMaximum=1.8384636640548706
  first_harmonic_tracker_phase_u : Subsystem
  first_harmonic_tracker_phase_v : Subsystem
  first_harmonic_tracker_phase_w : Subsystem
  gamma_hat : Outport  VectorParamsAs1DForOutWhenUnconnected=off
  omega_pu_hat : Outport  Port=2  VectorParamsAs1DForOutWhenUnconnected=off
  dqpll_uxi : Outport  Port=3  VectorParamsAs1DForOutWhenUnconnected=off
  dqpll_ueta : Outport  Port=4  VectorParamsAs1DForOutWhenUnconnected=off
  dqpll_state : Outport  Port=5  VectorParamsAs1DForOutWhenUnconnected=off
  wires:
  Step/1 -> Data Type Conversion3/1
  Constant/1 -> Data Type Conversion1/1
  Data Type Conversion3/1 -> C Caller/1
  Data Type Conversion2/1 -> C Caller/2
  Data Type Conversion4/1 -> C Caller/3
  Data Type Conversion5/1 -> C Caller/4
  Data Type Conversion1/1 -> C Caller/5
  C Caller/1 -> Bus Selector/1
  Bus Selector/1 -> Data Type Conversion6/1  "<omega_pu_hat>"
  Bus Selector/2 -> Data Type Conversion7/1  "<gamma_hat>"
  Bus Selector/3 -> Data Type Conversion8/1  "<u_grid_xi>"
  Bus Selector/4 -> Data Type Conversion9/1  "<u_grid_eta>"
  Bus Selector/5 -> Data Type Conversion10/1  "<dqpll_pll_state>"
  Data Type Conversion7/1 -> gamma_hat/1
  Data Type Conversion10/1 -> dqpll_state/1
  Data Type Conversion8/1 -> dqpll_uxi/1
  Data Type Conversion9/1 -> dqpll_ueta/1
  ug_abc_pu/1 -> Demux/1
  Demux/2 -> Quantizer1/1
  Demux/1 -> Quantizer2/1
  Demux/3 -> Quantizer4/1
  Quantizer2/1 -> Unit Delay2/1
  Unit Delay2/1 -> first_harmonic_tracker_phase_u/1(u)
  Unit Delay1/1 -> first_harmonic_tracker_phase_v/1(u)
  Unit Delay3/1 -> first_harmonic_tracker_phase_w/1(u)
  Quantizer1/1 -> Unit Delay1/1
  Quantizer4/1 -> Unit Delay3/1
  Data Type Conversion6/1 -> omega_pu_hat/1
  first_harmonic_tracker_phase_u/1(u_hat) -> first_harmonic_tracker/1, Data Type Conversion2/1  "tracker_phase_u"
  first_harmonic_tracker_phase_v/1(u_hat) -> first_harmonic_tracker/2, Data Type Conversion4/1  "tracker_phase_v"
  first_harmonic_tracker_phase_w/1(u_hat) -> first_harmonic_tracker/3, Data Type Conversion5/1  "tracker_phase_w"

== system afe_abc_inv_psm_2mods/afe_abc_inv_psm_mod1/AFE_control/afe_control/grid_voltage_sequences/grid_voltage_sampling_and_alpha_beta_transformation ==
  v_abc : Inport
  v_abc2alphabeta : MATLAB Function  TreatAsAtomicUnit=on
  u_grid_alpha : Outport
  u_grid_beta : Outport  Port=2
  wires:
  v_abc2alphabeta/1(alpha) -> u_grid_alpha/1  "u_grid_alpha"
  v_abc2alphabeta/2(beta) -> u_grid_beta/1  "u_grid_beta"
  v_abc/1 -> v_abc2alphabeta/1(v_abc)

== system afe_abc_inv_psm_2mods/afe_abc_inv_psm_mod1/AFE_control/afe_control/grid_voltage_sequences/v_alphabeta2xieta ==
  alpha : Inport
  beta : Inport  Port=2
  gamma : Inport  Port=3
  MATLAB Function : MATLAB Function  TreatAsAtomicUnit=on
  MATLAB Function1 : MATLAB Function  TreatAsAtomicUnit=on
  xi : Outport
  eta : Outport  Port=2
  v_grid_neg_xi : Outport  Port=3
  v_grid_neg_eta : Outport  Port=4
  wires:
  alpha/1 -> MATLAB Function1/1(alpha), MATLAB Function/1(alpha)  "u_grid_alpha"
  beta/1 -> MATLAB Function1/2(beta), MATLAB Function/2(beta)  "u_grid_beta"
  gamma/1 -> MATLAB Function1/3(gamma), MATLAB Function/3(gamma)  "gamma_grid"
  MATLAB Function/1(xi) -> xi/1  "u_grid_pos_xi"
  MATLAB Function/2(eta) -> eta/1  "u_grid_pos_eta"
  MATLAB Function1/1(xi) -> v_grid_neg_xi/1  "u_grid_neg_xi"
  MATLAB Function1/2(eta) -> v_grid_neg_eta/1  "u_grid_neg_eta"

== system afe_abc_inv_psm_2mods/afe_abc_inv_psm_mod1/AFE_control/afe_control/grid_voltage_sequences/voltage_sequence_avg ==
  v_grid_pos_xi : Inport
  v_grid_pos_eta : Inport  Port=2
  v_grid_neg_xi : Inport  Port=3
  v_grid_neg_eta : Inport  Port=4
  Variant Source{1..4} (4 alike) : VariantSource  VariantControls={use_moving_average_from_ccaller_mod1 == 1, use_moving_average_from_ccaller_mod1 == 0}
  average_filter_ccaller : Subsystem
  average_filter_simulink : Subsystem
  v_grid_pos_xi_avg : Outport
  v_grid_pos_eta_avg : Outport  Port=2
  v_grid_neg_xi_avg : Outport  Port=3
  v_grid_neg_eta_avg : Outport  Port=4
  wires:
  v_grid_pos_xi/1 -> average_filter_simulink/1(v_grid_pos_xi), average_filter_ccaller/1(v_grid_pos_xi)
  v_grid_pos_eta/1 -> average_filter_simulink/2(v_grid_pos_eta), average_filter_ccaller/2(v_grid_pos_eta)
  v_grid_neg_xi/1 -> average_filter_simulink/3(v_grid_neg_xi), average_filter_ccaller/3(v_grid_neg_xi)
  v_grid_neg_eta/1 -> average_filter_simulink/4(v_grid_neg_eta), average_filter_ccaller/4(v_grid_neg_eta)
  Variant Source4/1 -> v_grid_pos_xi_avg/1
  Variant Source1/1 -> v_grid_pos_eta_avg/1
  Variant Source2/1 -> v_grid_neg_xi_avg/1
  Variant Source3/1 -> v_grid_neg_eta_avg/1
  average_filter_ccaller/1(v_grid_pos_xi_avg) -> Variant Source4/1
  average_filter_ccaller/2(v_grid_pos_eta_avg) -> Variant Source1/1
  average_filter_ccaller/3(v_grid_neg_xi_avg) -> Variant Source2/1
  average_filter_ccaller/4(v_grid_neg_eta_avg) -> Variant Source3/1
  average_filter_simulink/1(v_grid_pos_xi_avg) -> Variant Source4/2
  average_filter_simulink/2(v_grid_pos_eta_avg) -> Variant Source1/2
  average_filter_simulink/3(v_grid_neg_xi_avg) -> Variant Source2/2
  average_filter_simulink/4(v_grid_neg_eta_avg) -> Variant Source3/2

== system afe_abc_inv_psm_2mods/afe_abc_inv_psm_mod1/AFE_control/afe_control/ig afe quantizzation and one step delay/ig afe quantizzation and one step delay ==
  ig_u_pu : Inport
  ig_v_pu : Inport  Port=2
  ig_w_pu : Inport  Port=3
  Gain4 : Gain  Gain=-1
  Gain5 : Gain  Gain=-1
  Gain6 : Gain  Gain=-1
  Quantizer1 : Quantizer  QuantizationInterval=adc_quantization
  Quantizer2 : Quantizer  QuantizationInterval=adc_quantization
  Quantizer4 : Quantizer  QuantizationInterval=adc_quantization
  Unit Delay : UnitDelay  SampleTime=-1  HasFrameUpgradeWarning=on
  Unit Delay1 : UnitDelay  SampleTime=-1  HasFrameUpgradeWarning=on
  Unit Delay2 : UnitDelay  SampleTime=-1  HasFrameUpgradeWarning=on
  igd_u_pu : Outport
  igd_v_pu : Outport  Port=2
  igd_w_pu : Outport  Port=3
  wires:
  Quantizer1/1 -> Unit Delay1/1
  Quantizer4/1 -> Unit Delay/1
  Quantizer2/1 -> Unit Delay2/1
  ig_u_pu/1 -> Quantizer4/1
  ig_v_pu/1 -> Quantizer1/1
  ig_w_pu/1 -> Quantizer2/1
  Unit Delay/1 -> Gain4/1
  Unit Delay1/1 -> Gain5/1
  Unit Delay2/1 -> Gain6/1
  Gain4/1 -> igd_u_pu/1
  Gain5/1 -> igd_v_pu/1
  Gain6/1 -> igd_w_pu/1

== system afe_abc_inv_psm_2mods/afe_abc_inv_psm_mod1/AFE_control/afe_control/instantaneus_power/abc2alphabeta ==
  a : Inport
  b : Inport  Port=2
  c : Inport  Port=3
  Gain1 : Gain  Gain=-1/2
  Gain11 : Gain  Gain=-1/2
  Gain2 : Gain  Gain=0
  Gain3 : Gain  Gain=sqrt(3)/2
  Gain4 : Gain  Gain=-sqrt(3)/2
  Gain8 : Gain  Gain=2/3
  Gain9 : Gain  Gain=2/3
  Sum : Sum  Inputs=+++
  Sum1 : Sum  Inputs=+++
  "alpha " : Outport  VectorParamsAs1DForOutWhenUnconnected=off
  "beta " : Outport  Port=2  VectorParamsAs1DForOutWhenUnconnected=off
  wires:
  Gain3/1 -> Sum1/2
  Gain2/1 -> Sum1/1
  Gain11/1 -> Sum/2
  Gain4/1 -> Sum1/3
  Sum1/1 -> Gain9/1
  Gain8/1 -> "alpha "/1
  Sum/1 -> Gain8/1
  c/1 -> Gain4/1, Gain1/1
  Gain9/1 -> "beta "/1
  b/1 -> Gain3/1, Gain11/1
  Gain1/1 -> Sum/3
  a/1 -> Gain2/1, Sum/1

== system afe_abc_inv_psm_2mods/afe_abc_inv_psm_mod1/AFE_control/afe_control/instantaneus_power/abc2alphabeta  ==
  a : Inport
  b : Inport  Port=2
  c : Inport  Port=3
  Gain1 : Gain  Gain=-1/2
  Gain11 : Gain  Gain=-1/2
  Gain2 : Gain  Gain=0
  Gain3 : Gain  Gain=sqrt(3)/2
  Gain4 : Gain  Gain=-sqrt(3)/2
  Gain8 : Gain  Gain=2/3
  Gain9 : Gain  Gain=2/3
  Sum : Sum  Inputs=+++
  Sum1 : Sum  Inputs=+++
  "alpha " : Outport  VectorParamsAs1DForOutWhenUnconnected=off
  "beta " : Outport  Port=2  VectorParamsAs1DForOutWhenUnconnected=off
  wires:
  a/1 -> Sum/1, Gain2/1
  Gain2/1 -> Sum1/1
  Gain9/1 -> "beta "/1
  Gain11/1 -> Sum/2
  c/1 -> Gain1/1, Gain4/1
  Sum/1 -> Gain8/1
  Sum1/1 -> Gain9/1
  Gain1/1 -> Sum/3
  Gain3/1 -> Sum1/2
  Gain4/1 -> Sum1/3
  Gain8/1 -> "alpha "/1
  b/1 -> Gain11/1, Gain3/1

== system afe_abc_inv_psm_2mods/afe_abc_inv_psm_mod1/AFE_control/afe_control/instantaneus_power/moving_avarage_p ==
  in : Inport
  Gain : Gain  Gain=n1-1
  Gain1 : Gain  Gain=1/n1
  Sum : Sum  Inputs=|++
  Unit Delay : UnitDelay  SampleTime=-1  HasFrameUpgradeWarning=on
  out : Outport  VectorParamsAs1DForOutWhenUnconnected=off
  wires:
  Gain/1 -> Sum/2
  Gain1/1 -> out/1, Unit Delay/1
  in/1 -> Sum/1
  Unit Delay/1 -> Gain/1
  Sum/1 -> Gain1/1

== system afe_abc_inv_psm_2mods/afe_abc_inv_psm_mod1/AFE_control/afe_control/instantaneus_power/moving_avarage_q ==
  in : Inport
  Gain : Gain  Gain=n1-1
  Gain1 : Gain  Gain=1/n1
  Sum : Sum  Inputs=|++
  Unit Delay : UnitDelay  SampleTime=-1  HasFrameUpgradeWarning=on
  out : Outport  VectorParamsAs1DForOutWhenUnconnected=off
  wires:
  Sum/1 -> Gain1/1
  Unit Delay/1 -> Gain/1
  in/1 -> Sum/1
  Gain1/1 -> Unit Delay/1, out/1
  Gain/1 -> Sum/2

== system afe_abc_inv_psm_2mods/afe_abc_inv_psm_mod1/AFE_control/afe_control/instantaneus_power/rms ==
  In1 : Inport
  Gain : Gain  Gain=n10-1
  Gain1 : Gain  Gain=1/n10
  Math Function : Math  Operator=magnitude^2  SignedPower=on
  Sqrt : Sqrt
  Sum : Sum  Inputs=|++
  Unit Delay : UnitDelay  SampleTime=-1  HasFrameUpgradeWarning=on
  Out1 : Outport  VectorParamsAs1DForOutWhenUnconnected=off
  wires:
  In1/1 -> Math Function/1
  Sum/1 -> Gain1/1
  Gain1/1 -> Sqrt/1, Unit Delay/1
  Unit Delay/1 -> Gain/1
  Math Function/1 -> Sum/1
  Sqrt/1 -> Out1/1
  Gain/1 -> Sum/2

== system afe_abc_inv_psm_2mods/afe_abc_inv_psm_mod1/AFE_control/afe_control/instantaneus_power/rms1 ==
  In1 : Inport
  Gain : Gain  Gain=n10-1
  Gain1 : Gain  Gain=1/n10
  Math Function : Math  Operator=magnitude^2  SignedPower=on
  Sqrt : Sqrt
  Sum : Sum  Inputs=|++
  Unit Delay : UnitDelay  SampleTime=-1  HasFrameUpgradeWarning=on
  Out1 : Outport  VectorParamsAs1DForOutWhenUnconnected=off
  wires:
  Gain/1 -> Sum/2
  Sqrt/1 -> Out1/1
  Math Function/1 -> Sum/1
  Unit Delay/1 -> Gain/1
  Gain1/1 -> Unit Delay/1, Sqrt/1
  Sum/1 -> Gain1/1
  In1/1 -> Math Function/1
